simulink library "ESTS_LNGSL"  (R2022a)
settings: Solver=VariableStepAuto  StartTime=0.0  StopTime=10.0  RelTol=1e-3
undefined symbols (not defined in the file): p_RadWhlDynFr_m, p_RadWhlDynRe_m
settings Model: Creator=blatak  LastModifiedBy=blatak

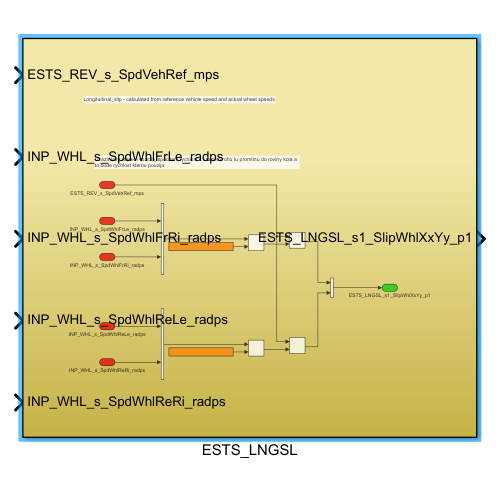
[thumbnail: Simulink's stored preview of the top-level diagram]
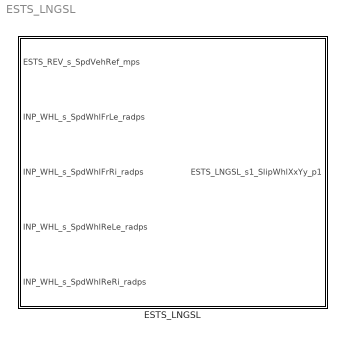
== system ESTS_LNGSL ==
  ESTS_LNGSL : Subsystem

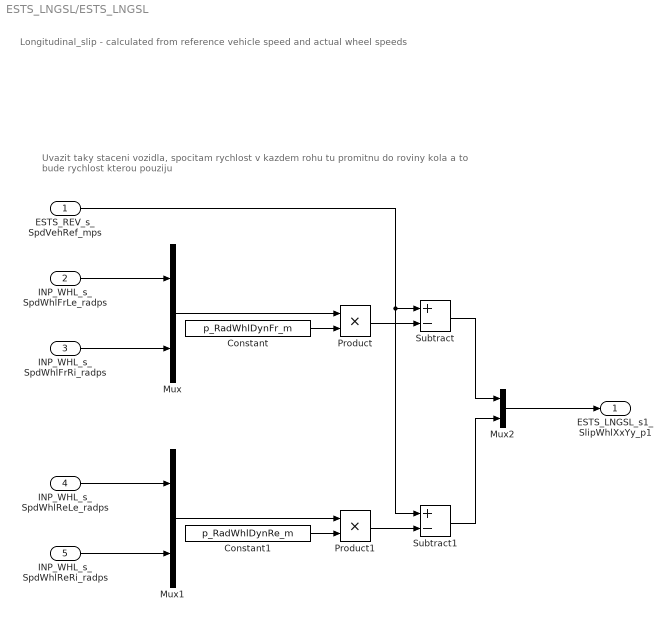
== system ESTS_LNGSL/ESTS_LNGSL ==
  note: Uvazit taky staceni vozidla, spocitam rychlost v kazdem rohu tu promitnu do roviny kola a to bude rychlost kterou pouziju
  note: Longitudinal_slip - calculated from reference vehicle speed and actual wheel speeds
  ESTS_REV_s_SpdVehRef_mps : Inport
  INP_WHL_s_SpdWhlFrLe_radps : Inport  Port=2
  INP_WHL_s_SpdWhlFrRi_radps : Inport  Port=3
  INP_WHL_s_SpdWhlReLe_radps : Inport  Port=4
  INP_WHL_s_SpdWhlReRi_radps : Inport  Port=5
  Constant : Constant  Value=p_RadWhlDynFr_m
  Constant1 : Constant  Value=p_RadWhlDynRe_m
  Mux : Mux  Inputs=2
  Mux1 : Mux  Inputs=2
  Mux2 : Mux  Inputs=2
  Product : Product
  Product1 : Product
  Subtract : Sum  Inputs=+-
  Subtract1 : Sum  Inputs=+-
  ESTS_LNGSL_s1_SlipWhlXxYy_p1 : Outport
  wires:
  INP_WHL_s_SpdWhlFrLe_radps/1 -> Mux/1
  INP_WHL_s_SpdWhlFrRi_radps/1 -> Mux/2
  INP_WHL_s_SpdWhlReRi_radps/1 -> Mux1/2
  INP_WHL_s_SpdWhlReLe_radps/1 -> Mux1/1
  Mux/1 -> Product/1
  Mux1/1 -> Product1/1
  Constant/1 -> Product/2
  Constant1/1 -> Product1/2
  Product/1 -> Subtract/2
  ESTS_REV_s_SpdVehRef_mps/1 -> Subtract1/1, Subtract/1
  Product1/1 -> Subtract1/2
  Subtract/1 -> Mux2/1
  Subtract1/1 -> Mux2/2
  Mux2/1 -> ESTS_LNGSL_s1_SlipWhlXxYy_p1/1
